simulink model "bh_CONCEPT_rate_limiter"  (R2016a)
settings: Solver=ode23t  StartTime=0.0  StopTime=5  FixedStep=0.001  RelTol=1e-5
settings Model: Creator=bhorton  LastModifiedBy=bhorton
settings DataIOCC: SaveOutput=off  SignalLogging=off  DSMLogging=off  VisualizeSimOutput=off  SaveTime=off
settings DebuggingCC: AllowSymbolicDim=off
settings ModelReferenceCC: PropagateSignalLabelsOutOfModel=off
settings GRTTargetCC: GeneratePreprocessorConditionals=Use local settings

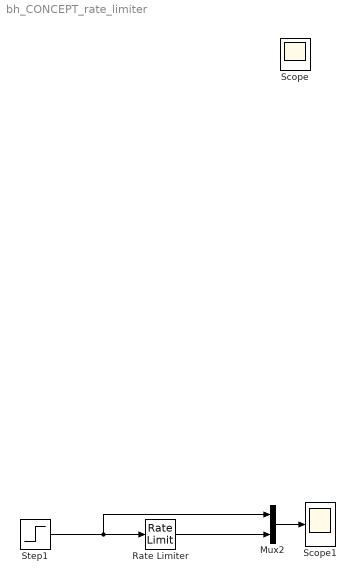
== system bh_CONCEPT_rate_limiter ==
  Mux2 : Mux  Inputs=2
  Rate Limiter : RateLimiter  RisingSlewLimit=5  FallingSlewLimit=-5
      settings: AttributesFormatString=|
      | Rising_rate = %<RisingSlewLimit>
      | Falling_rate = %<FallingSlewLimit>
  Scope1 : Scope
  Step1 : Step  Time=0.01  After=10  SampleTime=0
  Scope : Scope
  wires:
  Mux2/1 -> Scope1/1
  Step1/1 -> Mux2/1, Rate Limiter/1
  Rate Limiter/1 -> Mux2/2
